simulink model "UAV_formacao"  (R2024b)
settings: Solver=VariableStepAuto  StartTime=0.0  StopTime=tsim  RelTol=1e-3
values from neighbouring files (symbols this model uses):
  A = [ybb, yp+(w0/u0), yr-(u0/u0), g*cos(tt0)/u0 ... (first row only)    [init.m]    (also in new_A_B_integrativos.m = [A, zeros, zeros]; new_A_B_lambda.m = [A, zeros])
  B = [Yda, Ydr ... (first row only)    [init.m]    (also in new_A_B_integrativos.m = [B; new_line_bb; new_line_lambda]; new_A_B_lambda.m = [B; new_line_B])
  C = [0,1,0,0,0;0,0,1,0,0;-1,0,0,0,1;]    [main.m]    (also in untitled2.m = diag([1,1,1,1]))
  E0_f = P_f(1)    [main.m]
  E0_l = P_l(1)    [main.m]
  freq_amost = 100    [main.m]
  gg0 = 0    [Grupo3RP1.m]    (also in all_values.m; init.m; main.m; new_A_B_lambda.m)
  H = 0.44    [main.m]
  K = lqr(A_temp,B_temp,Q,R)    [K_lqr.m]    (also in k_finder.m = [0,0,0,0; main.m = K_lqr(A,B); untitled2.m = [0,0,0.229,0])
  L = lqe(A,G,C,Qe,Re)    [L_estim.m]    (also in k_finder.m = linspace(0,100,9999); main.m = L_estim(A,C))
  N0_f = P_f(2)    [main.m]
  N0_l = P_l(2)    [main.m]
  ref = [deg2rad(0), deg2rad(90)]    [main.m]
  sample_time = 1/freq_amost    (= 0.01)    [main.m]
  sample_time_gps = 1/freq_amos_gps    (= 0.2)    [main.m]
  t_slope = 10    [main.m]
  t_start = 20    [main.m]
  t_still = 50    [main.m]
  tt0 = gg0 + aa0    (= -3.65)    [Grupo3RP1.m]    (also in all_values.m; init.m; main.m; new_A_B_lambda.m)
  u0 = u0*0.51444    (= 27.985536)    [Grupo3RP1.m]    (also in all_values.m; init.m = [da0, dr0]; main.m; untitled2.m)
  Vwind = 3    [main.m]
  x0 = min(y_diff.signals.values)    [graficos_formacao.m]    (also in init.m = [0,0,0,0]; new_A_B_lambda.m = [0,0,0,0,0]')
libraries: simulink x24
settings Model: Creator=ruben  LastModifiedBy=quico
settings DataIOCC: ReturnWorkspaceOutputs=off

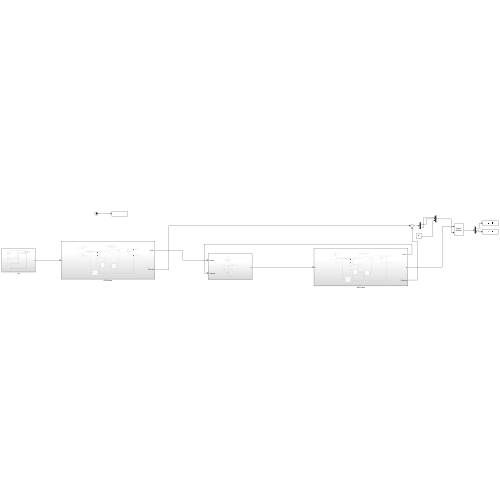
[thumbnail: Simulink's stored preview of the top-level diagram]
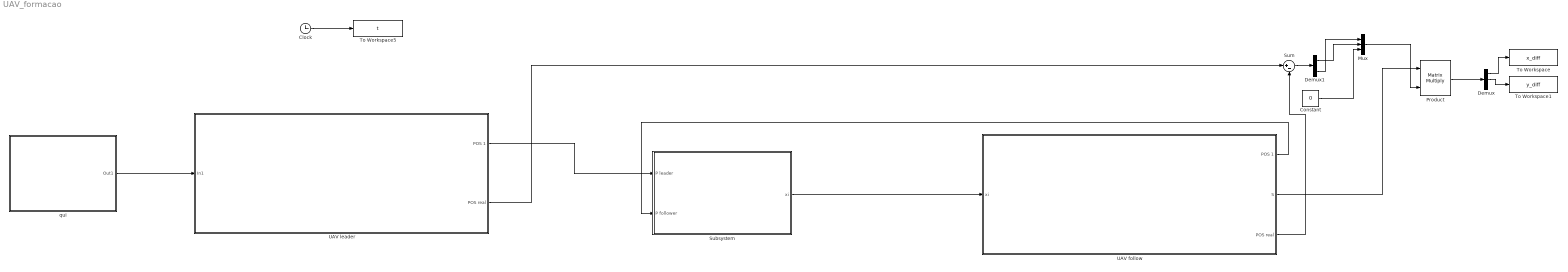
== system UAV_formacao ==
  " qui" : Subsystem
  Clock : Clock
  Constant : Constant  Value=0
  Demux : Demux  Outputs=3
  Demux1 : Demux  Outputs=2
  Mux : Mux  Inputs=3
  Product : Product  Multiplication=Matrix(*)
  Subsystem : Subsystem
  Sum : Sum  Inputs=|+-
  To Workspace : ToWorkspace  VariableName=x_diff  SaveFormat=Structure With Time  SampleTime=-1
  To Workspace1 : ToWorkspace  VariableName=y_diff  SaveFormat=Structure With Time  SampleTime=-1
  To Workspace5 : ToWorkspace  VariableName=t  SampleTime=-1
  UAV follow : Subsystem
  UAV leader : Subsystem
  wires:
  Clock/1 -> To Workspace5/1
  UAV leader/1(POS 1) -> Subsystem/1(P leader)
  UAV follow/1(POS 1) -> Subsystem/2(P follower)
  Subsystem/1(xi) -> UAV follow/1(xi)
  " qui"/1(Out1) -> UAV leader/1(In1)
  Product/1 -> Demux/1
  Demux/2 -> To Workspace1/1
  Demux/1 -> To Workspace/1
  Mux/1 -> Product/2
  UAV follow/2(S) -> Product/1
  Sum/1 -> Demux1/1
  Demux1/1 -> Mux/2
  Demux1/2 -> Mux/1
  Constant/1 -> Mux/3
  UAV leader/2(POS real) -> Sum/1
  UAV follow/3(POS real) -> Sum/2

== system UAV_formacao/ qui ==
  Ramp : simulink/Sources/Ramp  slope=ref(2)/t_slope  start=t_start  InitialOutput=0
  Ramp1 : simulink/Sources/Ramp  slope=-ref(2)/t_slope  start=t_start+t_slope  InitialOutput=0
  Ramp2 : simulink/Sources/Ramp  slope=-ref(2)/t_slope  start=t_start+t_slope+t_still  InitialOutput=0
  Ramp3 : simulink/Sources/Ramp  slope=ref(2)/t_slope  start=t_start+t_slope+t_still+t_slope  InitialOutput=0
  Sum1 : Sum  Inputs=|++++
  Out1 : Outport
  wires:
  Sum1/1 -> Out1/1
  Ramp/1 -> Sum1/1
  Ramp1/1 -> Sum1/2
  Ramp2/1 -> Sum1/3
  Ramp3/1 -> Sum1/4

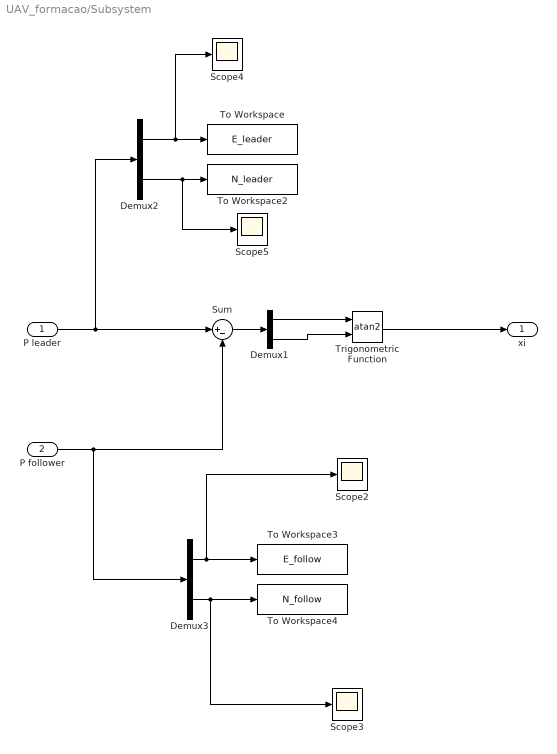
== system UAV_formacao/Subsystem ==
  P leader : Inport
  P follower : Inport  Port=2
  Demux1 : Demux  Outputs=2
  Demux2 : Demux  Outputs=2
  Demux3 : Demux  Outputs=2
  Scope{2..5} (4 alike) : Scope
  Sum : Sum  Inputs=|+-
  To Workspace : ToWorkspace  VariableName=E_leader  SaveFormat=Structure With Time  SampleTime=-1
  To Workspace2 : ToWorkspace  VariableName=N_leader  SaveFormat=Structure With Time  SampleTime=-1
  To Workspace3 : ToWorkspace  VariableName=E_follow  SaveFormat=Structure With Time  SampleTime=-1
  To Workspace4 : ToWorkspace  VariableName=N_follow  SaveFormat=Structure With Time  SampleTime=-1
  Trigonometric Function : Trigonometry  Operator=atan2
  xi : Outport
  wires:
  P leader/1 -> Demux2/1, Sum/1
  P follower/1 -> Demux3/1, Sum/2
  Demux2/1 -> Scope4/1, To Workspace/1
  Demux2/2 -> Scope5/1, To Workspace2/1
  Demux3/2 -> Scope3/1, To Workspace4/1
  Demux3/1 -> Scope2/1, To Workspace3/1
  Sum/1 -> Demux1/1
  Demux1/1 -> Trigonometric Function/1
  Demux1/2 -> Trigonometric Function/2
  Trigonometric Function/1 -> xi/1

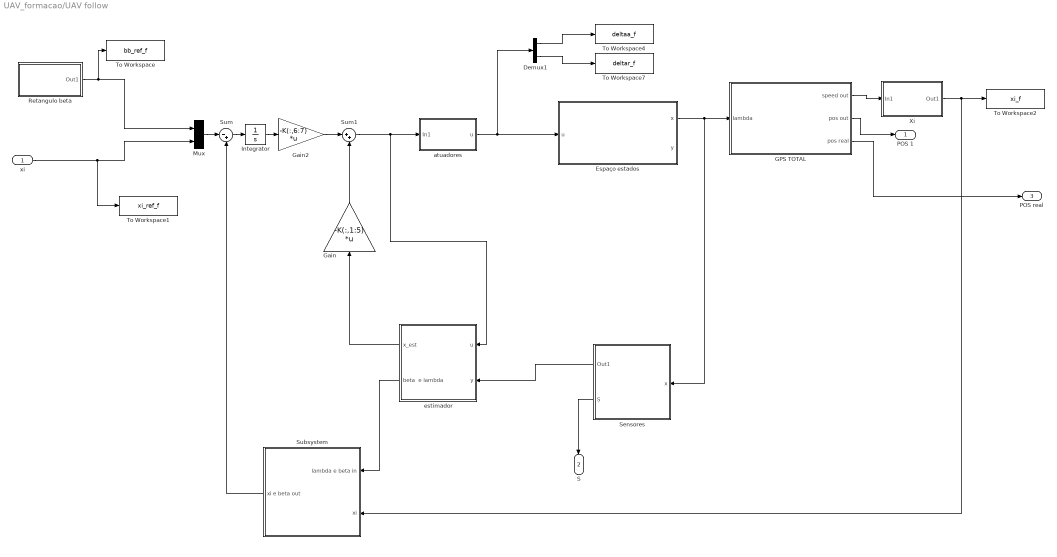
== system UAV_formacao/UAV follow ==
  xi : Inport
  Demux1 : Demux  Outputs=2
  Espaço estados : Subsystem
  GPS TOTAL : Subsystem
  Gain : Gain  Gain=-K(:,1:5)  Multiplication=Matrix(K*u)
  Gain2 : Gain  Gain=-K(:,6:7)  Multiplication=Matrix(K*u)
  Integrator : Integrator  InitialCondition=[0,0]
  Mux : Mux  Inputs=2
  Retangulo beta : Subsystem
  Sensores : Subsystem
  Subsystem : Subsystem
  Sum : Sum  Inputs=|-+
  Sum1 : Sum  Inputs=|++
  To Workspace : ToWorkspace  VariableName=bb_ref_f  SampleTime=-1
  To Workspace1 : ToWorkspace  VariableName=xi_ref_f  SampleTime=-1
  To Workspace2 : ToWorkspace  VariableName=xi_f  SaveFormat=Structure With Time  SampleTime=-1
  To Workspace4 : ToWorkspace  VariableName=deltaa_f  SampleTime=-1
  To Workspace7 : ToWorkspace  VariableName=deltar_f  SampleTime=-1
  Xi : Subsystem
  atuadores : Subsystem
  estimador : Subsystem
  POS 1 : Outport
  S : Outport  Port=2
  POS real : Outport  Port=3
  wires:
  Retangulo beta/1(Out1) -> To Workspace/1, Mux/1
  estimador/2(beta  e lambda) -> Subsystem/1(lambda e beta in)
  Gain/1 -> Sum1/2
  Sensores/1(Out1) -> estimador/2(y)
  estimador/1(x_est) -> Gain/1
  xi/1 -> To Workspace1/1, Mux/2
  Mux/1 -> Sum/1
  Sum/1 -> Integrator/1
  Integrator/1 -> Gain2/1
  Sum1/1 -> estimador/1(u), atuadores/1(In1)
  atuadores/1(u) -> Espaço estados/1(u), Demux1/1
  Subsystem/1(xi e beta out) -> Sum/2
  Gain2/1 -> Sum1/1
  Demux1/1 -> To Workspace4/1
  Demux1/2 -> To Workspace7/1
  GPS TOTAL/2(pos out) -> POS 1/1
  GPS TOTAL/1(speed out) -> Xi/1(In1)
  Xi/1(Out1) -> Subsystem/2(xi), To Workspace2/1
  Espaço estados/1(x) -> Sensores/1(x), GPS TOTAL/1(lambda)
  Sensores/2(S) -> S/1
  GPS TOTAL/3(pos real) -> POS real/1

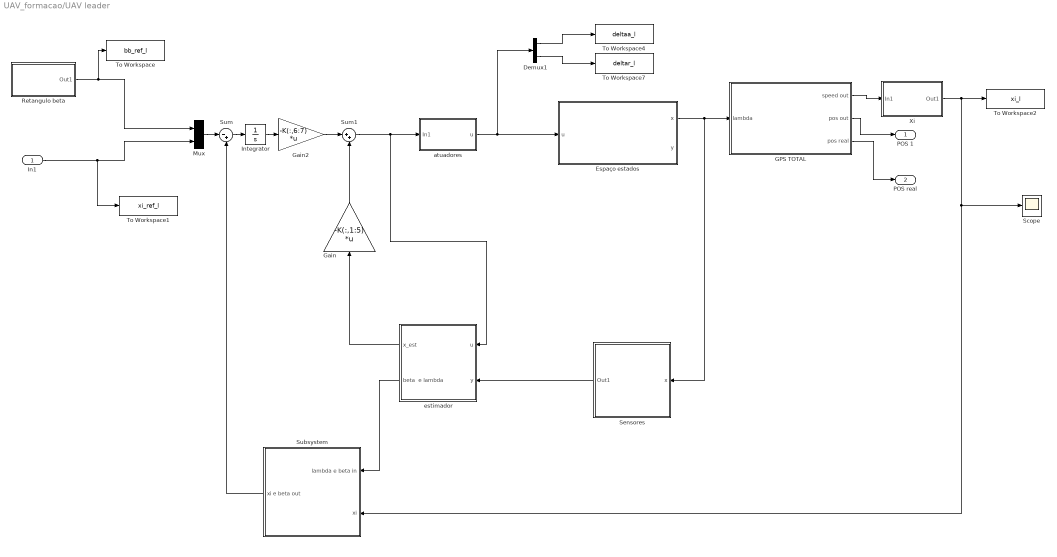
== system UAV_formacao/UAV leader ==
  In1 : Inport
  Demux1 : Demux  Outputs=2
  Espaço estados : Subsystem
  GPS TOTAL : Subsystem
  Gain : Gain  Gain=-K(:,1:5)  Multiplication=Matrix(K*u)
  Gain2 : Gain  Gain=-K(:,6:7)  Multiplication=Matrix(K*u)
  Integrator : Integrator  InitialCondition=[0,0]
  Mux : Mux  Inputs=2
  Retangulo beta : Subsystem
  Scope : Scope
  Sensores : Subsystem
  Subsystem : Subsystem
  Sum : Sum  Inputs=|-+
  Sum1 : Sum  Inputs=|++
  To Workspace : ToWorkspace  VariableName=bb_ref_l  SampleTime=-1
  To Workspace1 : ToWorkspace  VariableName=xi_ref_l  SampleTime=-1
  To Workspace2 : ToWorkspace  VariableName=xi_l  SaveFormat=Structure With Time  SampleTime=-1
  To Workspace4 : ToWorkspace  VariableName=deltaa_l  SampleTime=-1
  To Workspace7 : ToWorkspace  VariableName=deltar_l  SampleTime=-1
  Xi : Subsystem
  atuadores : Subsystem
  estimador : Subsystem
  POS 1 : Outport
  POS real : Outport  Port=2
  wires:
  Retangulo beta/1(Out1) -> To Workspace/1, Mux/1
  estimador/2(beta  e lambda) -> Subsystem/1(lambda e beta in)
  Gain/1 -> Sum1/2
  Sensores/1(Out1) -> estimador/2(y)
  estimador/1(x_est) -> Gain/1
  In1/1 -> To Workspace1/1, Mux/2
  Mux/1 -> Sum/1
  Sum/1 -> Integrator/1
  Integrator/1 -> Gain2/1
  Sum1/1 -> estimador/1(u), atuadores/1(In1)
  atuadores/1(u) -> Espaço estados/1(u), Demux1/1
  Subsystem/1(xi e beta out) -> Sum/2
  Gain2/1 -> Sum1/1
  Demux1/1 -> To Workspace4/1
  Demux1/2 -> To Workspace7/1
  GPS TOTAL/2(pos out) -> POS 1/1
  GPS TOTAL/1(speed out) -> Xi/1(In1)
  Xi/1(Out1) -> Scope/1, Subsystem/2(xi), To Workspace2/1
  Espaço estados/1(x) -> Sensores/1(x), GPS TOTAL/1(lambda)
  GPS TOTAL/3(pos real) -> POS real/1

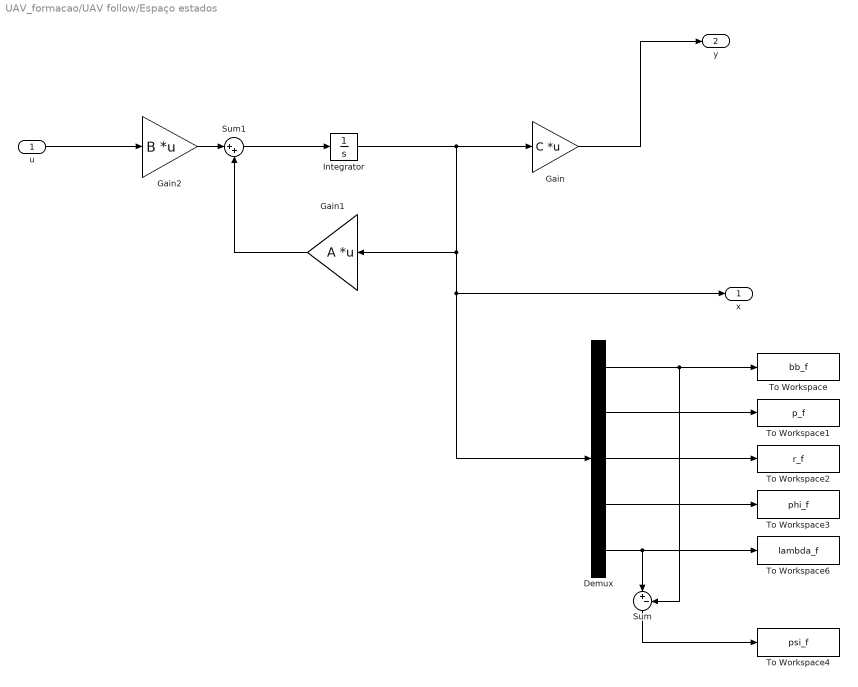
== system UAV_formacao/UAV follow/Espaço estados ==
  u : Inport
  Demux : Demux  Outputs=5
  Gain : Gain  Gain=C  Multiplication=Matrix(K*u)
  Gain1 : Gain  Gain=A  Multiplication=Matrix(K*u)
  Gain2 : Gain  Gain=B  Multiplication=Matrix(K*u)
  Integrator : Integrator  InitialCondition=x0
  Sum : Sum  Inputs=|+-
  Sum1 : Sum  Inputs=|++
  To Workspace : ToWorkspace  VariableName=bb_f  SampleTime=-1
  To Workspace1 : ToWorkspace  VariableName=p_f  SampleTime=-1
  To Workspace2 : ToWorkspace  VariableName=r_f  SampleTime=-1
  To Workspace3 : ToWorkspace  VariableName=phi_f  SampleTime=-1
  To Workspace4 : ToWorkspace  VariableName=psi_f  SampleTime=-1
  To Workspace6 : ToWorkspace  VariableName=lambda_f  SampleTime=-1
  x : Outport
  y : Outport  Port=2
  wires:
  u/1 -> Gain2/1
  Sum1/1 -> Integrator/1
  Demux/4 -> To Workspace3/1
  Demux/3 -> To Workspace2/1
  Demux/1 -> Sum/2, To Workspace/1
  Demux/2 -> To Workspace1/1
  Demux/5 -> Sum/1, To Workspace6/1
  Gain2/1 -> Sum1/1
  Integrator/1 -> Gain1/1, x/1, Demux/1, Gain/1
  Gain1/1 -> Sum1/2
  Gain/1 -> y/1
  Sum/1 -> To Workspace4/1

== system UAV_formacao/UAV follow/GPS TOTAL ==
  lambda : Inport
  Cinematica : Subsystem
  GPS : Subsystem
  speed out : Outport
  pos out : Outport  Port=2
  pos real : Outport  Port=3
  wires:
  Cinematica/2(pos) -> pos real/1, GPS/2(pos)
  GPS/2(pos out) -> pos out/1
  Cinematica/1(speed) -> GPS/1(speed)
  lambda/1 -> Cinematica/1(lambda)
  GPS/1(speed out) -> speed out/1

== system UAV_formacao/UAV follow/Retangulo beta ==
  Sum1 : Sum  Inputs=|++
  beta : Step  Time=25  After=-ref(1)  SampleTime=0
  beta_1 : Step  Time=10  After=ref(1)  SampleTime=0
  Out1 : Outport
  wires:
  beta/1 -> Sum1/1
  beta_1/1 -> Sum1/2
  Sum1/1 -> Out1/1

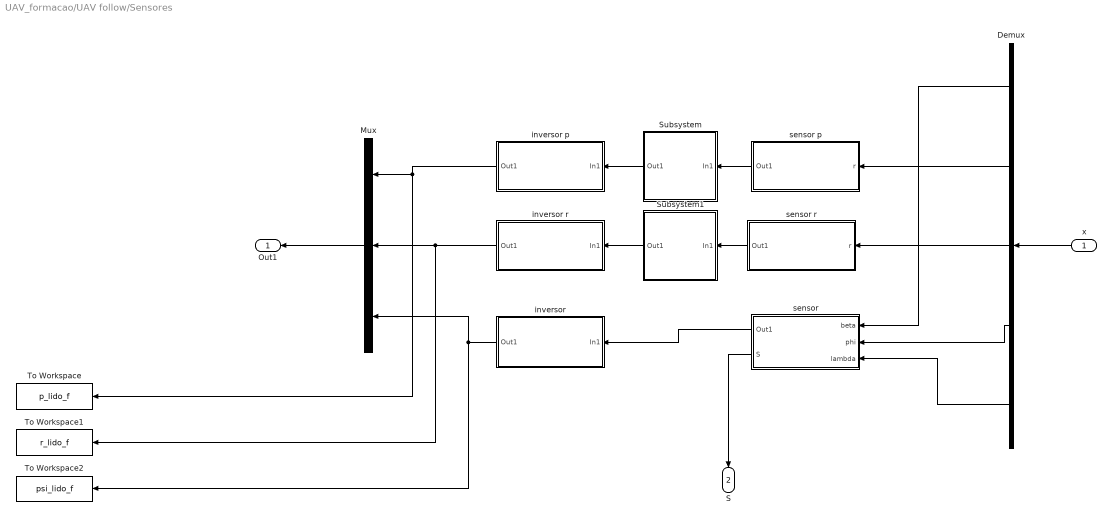
== system UAV_formacao/UAV follow/Sensores ==
  x : Inport
  Demux : Demux  Outputs=5
  Mux : Mux  Inputs=3
  Subsystem : Subsystem
  Subsystem1 : Subsystem
  To Workspace : ToWorkspace  VariableName=p_lido_f  SampleTime=-1
  To Workspace1 : ToWorkspace  VariableName=r_lido_f  SampleTime=-1
  To Workspace2 : ToWorkspace  VariableName=psi_lido_f  SampleTime=-1
  inversor : Subsystem
  inversor p : Subsystem
  inversor r : Subsystem
  sensor : Subsystem
  sensor p : Subsystem
  sensor r : Subsystem
  Out1 : Outport
  S : Outport  Port=2
  wires:
  inversor p/1(Out1) -> To Workspace/1, Mux/1
  Mux/1 -> Out1/1
  inversor r/1(Out1) -> To Workspace1/1, Mux/2
  x/1 -> Demux/1
  sensor/1(Out1) -> inversor/1(In1)
  inversor/1(Out1) -> To Workspace2/1, Mux/3
  Demux/2 -> sensor p/1(r)
  Demux/3 -> sensor r/1(r)
  Demux/1 -> sensor/1(beta)
  Demux/4 -> sensor/2(phi)
  Demux/5 -> sensor/3(lambda)
  Subsystem1/1(Out1) -> inversor r/1(In1)
  sensor r/1(Out1) -> Subsystem1/1(In1)
  sensor p/1(Out1) -> Subsystem/1(In1)
  Subsystem/1(Out1) -> inversor p/1(In1)
  sensor/2(S) -> S/1

== system UAV_formacao/UAV follow/Subsystem ==
  lambda e beta in : Inport
  xi : Inport  Port=2
  Demux : Demux  Outputs=2
  Mux1 : Mux  Inputs=2
  Sum2 : Sum  Inputs=|-+
  Sum3 : Sum  Inputs=|++
  xi e beta out : Outport
  wires:
  xi/1 -> Sum2/2
  Sum3/1 -> Mux1/2
  Demux/1 -> Mux1/1
  Mux1/1 -> xi e beta out/1
  lambda e beta in/1 -> Demux/1
  Demux/2 -> Sum2/1, Sum3/1
  Sum2/1 -> Sum3/2

== system UAV_formacao/UAV follow/Xi ==
  In1 : Inport
  Demux : Demux  Outputs=2
  Trigonometric Function : Trigonometry  Operator=atan2
  Out1 : Outport
  wires:
  Demux/1 -> Trigonometric Function/2
  Demux/2 -> Trigonometric Function/1
  Trigonometric Function/1 -> Out1/1
  In1/1 -> Demux/1

== system UAV_formacao/UAV follow/atuadores ==
  In1 : Inport
  Demux : Demux  Outputs=2
  Mux : Mux  Inputs=2
  Rate Limiter : RateLimiter  SampleTimeMode=inherited
  Rate Limiter1 : RateLimiter  SampleTimeMode=inherited
  Saturation : Saturate  UpperLimit=30*pi/180  LowerLimit=-30*pi/180
  Saturation1 : Saturate  UpperLimit=30*pi/180  LowerLimit=-30*pi/180
  Transfer Fcn : TransferFcn  Denominator=[0.04 1]
  Transfer Fcn1 : TransferFcn  Denominator=[0.04 1]
  Zero-Order Hold : ZeroOrderHold  SampleTime=1/100
  Zero-Order Hold1 : ZeroOrderHold  SampleTime=1/100
  u : Outport
  wires:
  In1/1 -> Demux/1
  Mux/1 -> u/1
  Demux/1 -> Zero-Order Hold/1  "deltaa"
  Demux/2 -> Zero-Order Hold1/1  "deltar"
  Transfer Fcn1/1 -> Mux/2
  Transfer Fcn/1 -> Mux/1
  Rate Limiter/1 -> Transfer Fcn/1
  Rate Limiter1/1 -> Transfer Fcn1/1
  Saturation1/1 -> Rate Limiter1/1
  Saturation/1 -> Rate Limiter/1
  Zero-Order Hold/1 -> Saturation/1
  Zero-Order Hold1/1 -> Saturation1/1

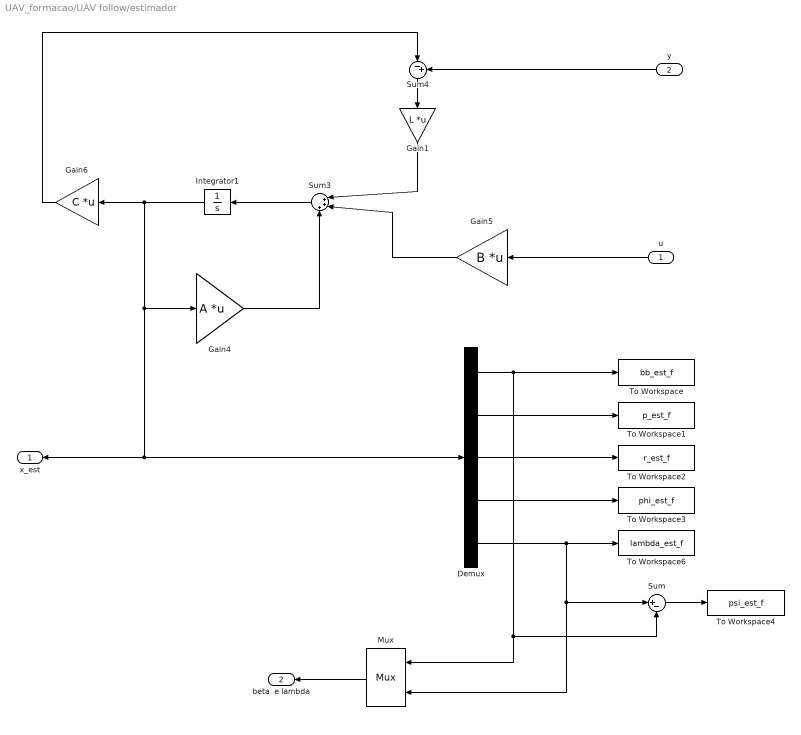
== system UAV_formacao/UAV follow/estimador ==
  u : Inport
  y : Inport  Port=2
  Demux : Demux  Outputs=5
  Gain1 : Gain  Gain=L  Multiplication=Matrix(K*u)
  Gain4 : Gain  Gain=A  Multiplication=Matrix(K*u)
  Gain5 : Gain  Gain=B  Multiplication=Matrix(K*u)
  Gain6 : Gain  Gain=C  Multiplication=Matrix(K*u)
  Integrator1 : Integrator  InitialCondition=x0
  Mux : Mux  Inputs=2
      settings: DisplayOption=signals
  Sum : Sum  Inputs=|+-
  Sum3 : Sum  Inputs=|+++
  Sum4 : Sum  Inputs=|-+
  To Workspace : ToWorkspace  VariableName=bb_est_f  SampleTime=-1
  To Workspace1 : ToWorkspace  VariableName=p_est_f  SampleTime=-1
  To Workspace2 : ToWorkspace  VariableName=r_est_f  SampleTime=-1
  To Workspace3 : ToWorkspace  VariableName=phi_est_f  SampleTime=-1
  To Workspace4 : ToWorkspace  VariableName=psi_est_f  SampleTime=-1
  To Workspace6 : ToWorkspace  VariableName=lambda_est_f  SampleTime=-1
  x_est : Outport
  beta  e lambda : Outport  Port=2
  wires:
  Demux/5 -> Sum/1, Mux/2, To Workspace6/1
  Demux/2 -> To Workspace1/1
  Demux/3 -> To Workspace2/1
  Demux/4 -> To Workspace3/1
  Demux/1 -> Sum/2, Mux/1, To Workspace/1
  Integrator1/1 -> Demux/1, x_est/1, Gain4/1, Gain6/1
  Sum3/1 -> Integrator1/1
  u/1 -> Gain5/1
  Gain4/1 -> Sum3/3
  y/1 -> Sum4/2
  Gain6/1 -> Sum4/1
  Gain5/1 -> Sum3/2
  Mux/1 -> beta  e lambda/1
  Sum4/1 -> Gain1/1
  Gain1/1 -> Sum3/1
  Sum/1 -> To Workspace4/1

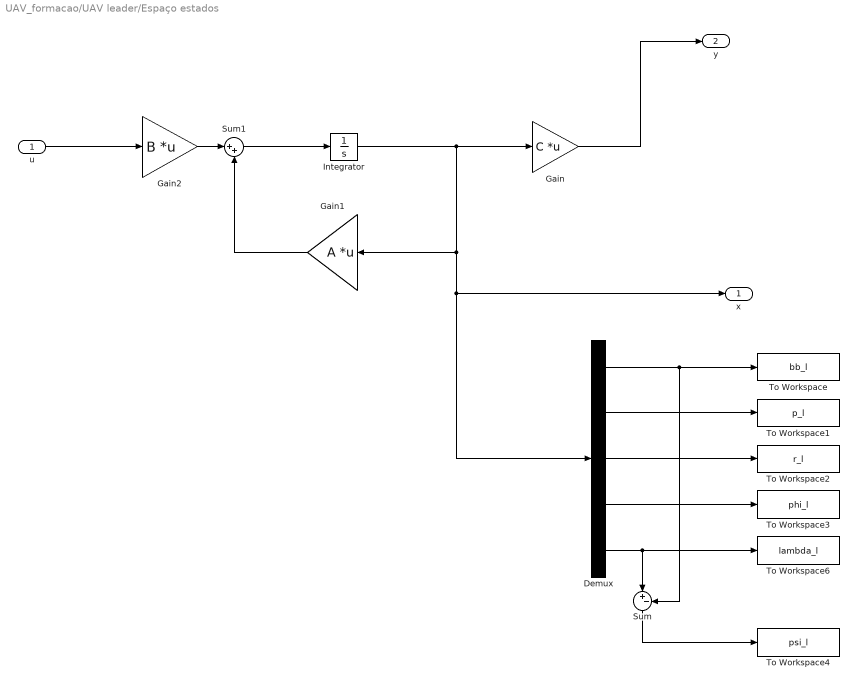
== system UAV_formacao/UAV leader/Espaço estados ==
  u : Inport
  Demux : Demux  Outputs=5
  Gain : Gain  Gain=C  Multiplication=Matrix(K*u)
  Gain1 : Gain  Gain=A  Multiplication=Matrix(K*u)
  Gain2 : Gain  Gain=B  Multiplication=Matrix(K*u)
  Integrator : Integrator  InitialCondition=x0
  Sum : Sum  Inputs=|+-
  Sum1 : Sum  Inputs=|++
  To Workspace : ToWorkspace  VariableName=bb_l  SampleTime=-1
  To Workspace1 : ToWorkspace  VariableName=p_l  SampleTime=-1
  To Workspace2 : ToWorkspace  VariableName=r_l  SampleTime=-1
  To Workspace3 : ToWorkspace  VariableName=phi_l  SampleTime=-1
  To Workspace4 : ToWorkspace  VariableName=psi_l  SampleTime=-1
  To Workspace6 : ToWorkspace  VariableName=lambda_l  SampleTime=-1
  x : Outport
  y : Outport  Port=2
  wires:
  u/1 -> Gain2/1
  Sum1/1 -> Integrator/1
  Demux/4 -> To Workspace3/1
  Demux/3 -> To Workspace2/1
  Demux/1 -> Sum/2, To Workspace/1
  Demux/2 -> To Workspace1/1
  Demux/5 -> Sum/1, To Workspace6/1
  Gain2/1 -> Sum1/1
  Integrator/1 -> Gain1/1, x/1, Demux/1, Gain/1
  Gain1/1 -> Sum1/2
  Gain/1 -> y/1
  Sum/1 -> To Workspace4/1

== system UAV_formacao/UAV leader/GPS TOTAL ==
  lambda : Inport
  Cinematica : Subsystem
  GPS : Subsystem
  speed out : Outport
  pos out : Outport  Port=2
  pos real : Outport  Port=3
  wires:
  Cinematica/2(pos) -> pos real/1, GPS/2(pos)
  GPS/2(pos out) -> pos out/1
  Cinematica/1(speed) -> GPS/1(speed)
  lambda/1 -> Cinematica/1(lambda)
  GPS/1(speed out) -> speed out/1

== system UAV_formacao/UAV leader/Retangulo beta ==
  Sum1 : Sum  Inputs=|++
  beta : Step  Time=25  After=-ref(1)  SampleTime=0
  beta_1 : Step  Time=10  After=ref(1)  SampleTime=0
  Out1 : Outport
  wires:
  beta/1 -> Sum1/1
  beta_1/1 -> Sum1/2
  Sum1/1 -> Out1/1

== system UAV_formacao/UAV leader/Sensores ==
  x : Inport
  Demux : Demux  Outputs=5
  Mux : Mux  Inputs=3
  Subsystem : Subsystem
  Subsystem1 : Subsystem
  To Workspace : ToWorkspace  VariableName=p_lido_l  SampleTime=-1
  To Workspace1 : ToWorkspace  VariableName=r_lido_l  SampleTime=-1
  To Workspace2 : ToWorkspace  VariableName=psi_lido_l  SampleTime=-1
  inversor : Subsystem
  inversor p : Subsystem
  inversor r : Subsystem
  sensor : Subsystem
  sensor p : Subsystem
  sensor r : Subsystem
  Out1 : Outport
  wires:
  inversor p/1(Out1) -> To Workspace/1, Mux/1
  Mux/1 -> Out1/1
  inversor r/1(Out1) -> To Workspace1/1, Mux/2
  x/1 -> Demux/1
  sensor/1(Out1) -> inversor/1(In1)
  inversor/1(Out1) -> To Workspace2/1, Mux/3
  Demux/2 -> sensor p/1(r)
  Demux/3 -> sensor r/1(r)
  Demux/1 -> sensor/1(beta)
  Demux/4 -> sensor/2(phi)
  Demux/5 -> sensor/3(lambda)
  Subsystem1/1(Out1) -> inversor r/1(In1)
  sensor r/1(Out1) -> Subsystem1/1(In1)
  sensor p/1(Out1) -> Subsystem/1(In1)
  Subsystem/1(Out1) -> inversor p/1(In1)

== system UAV_formacao/UAV leader/Subsystem ==
  lambda e beta in : Inport
  xi : Inport  Port=2
  Demux : Demux  Outputs=2
  Mux1 : Mux  Inputs=2
  Sum2 : Sum  Inputs=|-+
  Sum3 : Sum  Inputs=|++
  xi e beta out : Outport
  wires:
  xi/1 -> Sum2/2
  Sum3/1 -> Mux1/2
  Demux/1 -> Mux1/1
  Mux1/1 -> xi e beta out/1
  lambda e beta in/1 -> Demux/1
  Demux/2 -> Sum2/1, Sum3/1
  Sum2/1 -> Sum3/2

== system UAV_formacao/UAV leader/Xi ==
  In1 : Inport
  Demux : Demux  Outputs=2
  Trigonometric Function : Trigonometry  Operator=atan2
  Out1 : Outport
  wires:
  Demux/1 -> Trigonometric Function/2
  Demux/2 -> Trigonometric Function/1
  Trigonometric Function/1 -> Out1/1
  In1/1 -> Demux/1

== system UAV_formacao/UAV leader/atuadores ==
  In1 : Inport
  Demux : Demux  Outputs=2
  Mux : Mux  Inputs=2
  Rate Limiter : RateLimiter  SampleTimeMode=inherited
  Rate Limiter1 : RateLimiter  SampleTimeMode=inherited
  Saturation : Saturate  UpperLimit=30*pi/180  LowerLimit=-30*pi/180
  Saturation1 : Saturate  UpperLimit=30*pi/180  LowerLimit=-30*pi/180
  Transfer Fcn : TransferFcn  Denominator=[0.04 1]
  Transfer Fcn1 : TransferFcn  Denominator=[0.04 1]
  Zero-Order Hold : ZeroOrderHold  SampleTime=1/100
  Zero-Order Hold1 : ZeroOrderHold  SampleTime=1/100
  u : Outport
  wires:
  In1/1 -> Demux/1
  Mux/1 -> u/1
  Demux/1 -> Zero-Order Hold/1  "deltaa"
  Demux/2 -> Zero-Order Hold1/1  "deltar"
  Transfer Fcn1/1 -> Mux/2
  Transfer Fcn/1 -> Mux/1
  Rate Limiter/1 -> Transfer Fcn/1
  Rate Limiter1/1 -> Transfer Fcn1/1
  Saturation1/1 -> Rate Limiter1/1
  Saturation/1 -> Rate Limiter/1
  Zero-Order Hold/1 -> Saturation/1
  Zero-Order Hold1/1 -> Saturation1/1

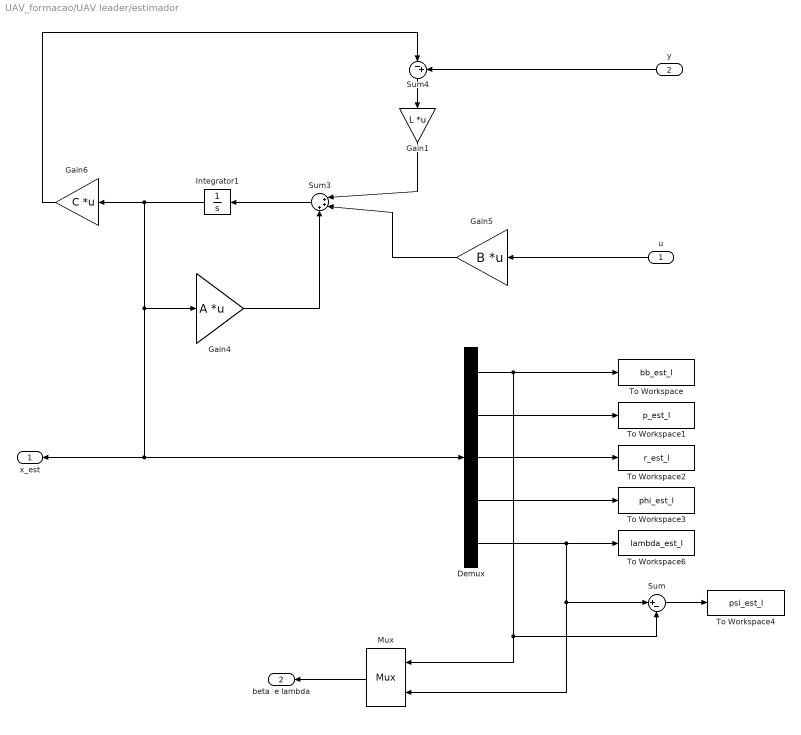
== system UAV_formacao/UAV leader/estimador ==
  u : Inport
  y : Inport  Port=2
  Demux : Demux  Outputs=5
  Gain1 : Gain  Gain=L  Multiplication=Matrix(K*u)
  Gain4 : Gain  Gain=A  Multiplication=Matrix(K*u)
  Gain5 : Gain  Gain=B  Multiplication=Matrix(K*u)
  Gain6 : Gain  Gain=C  Multiplication=Matrix(K*u)
  Integrator1 : Integrator  InitialCondition=x0
  Mux : Mux  Inputs=2
      settings: DisplayOption=signals
  Sum : Sum  Inputs=|+-
  Sum3 : Sum  Inputs=|+++
  Sum4 : Sum  Inputs=|-+
  To Workspace : ToWorkspace  VariableName=bb_est_l  SampleTime=-1
  To Workspace1 : ToWorkspace  VariableName=p_est_l  SampleTime=-1
  To Workspace2 : ToWorkspace  VariableName=r_est_l  SampleTime=-1
  To Workspace3 : ToWorkspace  VariableName=phi_est_l  SampleTime=-1
  To Workspace4 : ToWorkspace  VariableName=psi_est_l  SampleTime=-1
  To Workspace6 : ToWorkspace  VariableName=lambda_est_l  SampleTime=-1
  x_est : Outport
  beta  e lambda : Outport  Port=2
  wires:
  Demux/5 -> Sum/1, Mux/2, To Workspace6/1
  Demux/2 -> To Workspace1/1
  Demux/3 -> To Workspace2/1
  Demux/4 -> To Workspace3/1
  Demux/1 -> Sum/2, Mux/1, To Workspace/1
  Integrator1/1 -> Demux/1, x_est/1, Gain4/1, Gain6/1
  Sum3/1 -> Integrator1/1
  u/1 -> Gain5/1
  Gain4/1 -> Sum3/3
  y/1 -> Sum4/2
  Gain6/1 -> Sum4/1
  Gain5/1 -> Sum3/2
  Mux/1 -> beta  e lambda/1
  Sum4/1 -> Gain1/1
  Gain1/1 -> Sum3/1
  Sum/1 -> To Workspace4/1

== system UAV_formacao/UAV follow/GPS TOTAL/Cinematica ==
  lambda : Inport
  Constant1 : Constant  Value=gg0
  Constant2 : Constant  Value=u0
  Constant3 : Constant  Value=Vwind
  Demux : Demux  Outputs=5
  Integrator : Integrator  InitialCondition=E0_f
  Integrator1 : Integrator  InitialCondition=N0_f
  Mux1 : Mux  Inputs=2
  Mux2 : Mux  Inputs=2
  Product2 : Product
  Product3 : Product
  Subsystem : Subsystem
  Subsystem1 : Subsystem
  Sum : Sum  Inputs=|+-
  speed : Outport
  pos : Outport  Port=2
  wires:
  Constant2/1 -> Product3/2, Product2/1
  Product3/1 -> Mux2/2, Integrator/1
  Product2/1 -> Sum/1
  Constant3/1 -> Sum/2
  Sum/1 -> Mux2/1, Integrator1/1
  Integrator/1 -> Mux1/1
  Integrator1/1 -> Mux1/2
  Mux2/1 -> speed/1
  Mux1/1 -> pos/1
  Subsystem/1(Out1) -> Product3/1
  Constant1/1 -> Subsystem/2(In2), Subsystem1/1(In2)
  Subsystem1/1(Out1) -> Product2/2
  lambda/1 -> Demux/1
  Demux/5 -> Subsystem/1(In1), Subsystem1/2(In1)

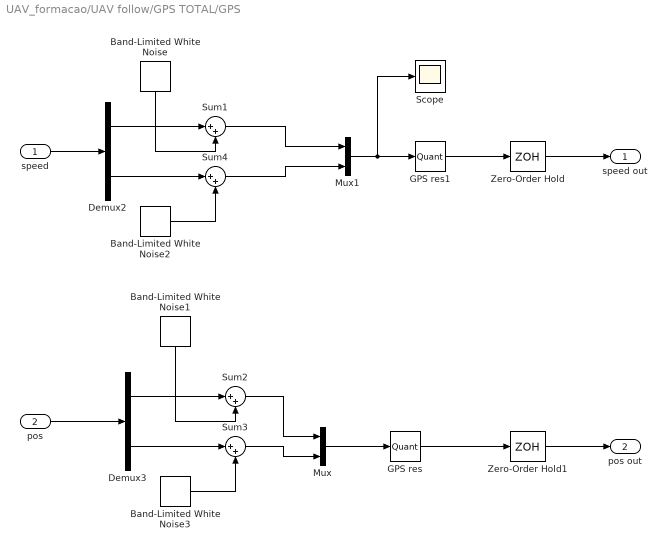
== system UAV_formacao/UAV follow/GPS TOTAL/GPS ==
  speed : Inport
  pos : Inport  Port=2
  Band-Limited White Noise : simulink/Sources/Band-Limited White Noise  Cov=sample_time_gps*0.1*0.1  Ts=sample_time_gps  seed=[13]
  Band-Limited White Noise1 : simulink/Sources/Band-Limited White Noise  Cov=sample_time_gps*2.5*2.5  Ts=sample_time_gps  seed=[15]
  Band-Limited White Noise2 : simulink/Sources/Band-Limited White Noise  Cov=sample_time_gps*0.1*0.1  Ts=sample_time_gps  seed=[14]
  Band-Limited White Noise3 : simulink/Sources/Band-Limited White Noise  Cov=sample_time_gps*2.5*2.5  Ts=sample_time_gps  seed=[16]
  Demux2 : Demux  Outputs=2
  Demux3 : Demux  Outputs=2
  GPS res : Quantizer
  GPS res1 : Quantizer  QuantizationInterval=0.01
  Mux : Mux  Inputs=2
  Mux1 : Mux  Inputs=2
  Scope : Scope
  Sum{1..4} (4 alike) : Sum  Inputs=|++
  Zero-Order Hold : ZeroOrderHold  SampleTime=sample_time_gps
  Zero-Order Hold1 : ZeroOrderHold  SampleTime=sample_time_gps
  speed out : Outport
  pos out : Outport  Port=2
  wires:
  Mux/1 -> GPS res/1
  GPS res/1 -> Zero-Order Hold1/1
  GPS res1/1 -> Zero-Order Hold/1
  Mux1/1 -> Scope/1, GPS res1/1
  speed/1 -> Demux2/1
  Demux2/1 -> Sum1/1
  Demux2/2 -> Sum4/1
  Band-Limited White Noise/1 -> Sum1/2
  Band-Limited White Noise2/1 -> Sum4/2
  Demux3/2 -> Sum3/1
  pos/1 -> Demux3/1
  Band-Limited White Noise3/1 -> Sum3/2
  Demux3/1 -> Sum2/1
  Band-Limited White Noise1/1 -> Sum2/2
  Sum2/1 -> Mux/1
  Sum3/1 -> Mux/2
  Sum4/1 -> Mux1/2
  Sum1/1 -> Mux1/1
  Zero-Order Hold/1 -> speed out/1
  Zero-Order Hold1/1 -> pos out/1

== system UAV_formacao/UAV follow/Sensores/Subsystem ==
  In1 : Inport
  Band-Limited White Noise : simulink/Sources/Band-Limited White Noise  Cov=[sample_time*(2*(5/(2^12)))^2]  Ts=sample_time  seed=[1]
  Quantizer : Quantizer  QuantizationInterval=5/(2^12)
  Saturation : Saturate  UpperLimit=5  LowerLimit=0
  Sum : Sum  Inputs=|++
  Out1 : Outport
  wires:
  In1/1 -> Sum/1
  Saturation/1 -> Out1/1
  Band-Limited White Noise/1 -> Sum/2
  Quantizer/1 -> Saturation/1
  Sum/1 -> Quantizer/1

== system UAV_formacao/UAV follow/Sensores/Subsystem1 ==
  In1 : Inport
  Band-Limited White Noise : simulink/Sources/Band-Limited White Noise  Cov=[sample_time*(2*(5/(2^12)))^2]  Ts=sample_time  seed=[2]
  Quantizer : Quantizer  QuantizationInterval=5/(2^12)
  Saturation : Saturate  UpperLimit=5  LowerLimit=0
  Sum : Sum  Inputs=|++
  Out1 : Outport
  wires:
  In1/1 -> Sum/1
  Saturation/1 -> Out1/1
  Band-Limited White Noise/1 -> Sum/2
  Quantizer/1 -> Saturation/1
  Sum/1 -> Quantizer/1

== system UAV_formacao/UAV follow/Sensores/inversor ==
  In1 : Inport
  Band-Limited White Noise1 : simulink/Sources/Band-Limited White Noise  Cov=[0.005*0.005*freq_amost]  Ts=freq_amost  seed=[11]
  Band-Limited White Noise2 : simulink/Sources/Band-Limited White Noise  Cov=[0.005*0.005*sample_time]  Ts=sample_time  seed=[12]
  Demux : Demux  Outputs=3
  Gain : Gain  Gain=-1
  Quantizer : Quantizer  QuantizationInterval=0.005
  Quantizer1 : Quantizer  QuantizationInterval=0.005
  Saturation : Saturate  UpperLimit=8  LowerLimit=-8
  Saturation1 : Saturate  UpperLimit=8  LowerLimit=-8
  Sum : Sum  Inputs=|++
  Sum1 : Sum  Inputs=|++
  Trigonometric Function : Trigonometry  Operator=atan2
  Out1 : Outport
  wires:
  Band-Limited White Noise1/1 -> Sum/2
  Band-Limited White Noise2/1 -> Sum1/2
  Sum/1 -> Quantizer/1
  Sum1/1 -> Quantizer1/1
  Demux/1 -> Sum/1
  Trigonometric Function/1 -> Out1/1
  In1/1 -> Demux/1
  Demux/2 -> Sum1/1
  Gain/1 -> Trigonometric Function/1
  Saturation1/1 -> Gain/1
  Quantizer1/1 -> Saturation1/1
  Quantizer/1 -> Saturation/1
  Saturation/1 -> Trigonometric Function/2

== system UAV_formacao/UAV follow/Sensores/inversor p ==
  In1 : Inport
  Constant : Constant  Value=-1250/3
  Gain3 : Gain  Gain=(300-(-300))/(4.3-0.7)
  Gain5 : Gain  Gain=pi/180
  Sum : Sum  Inputs=|++
  Out1 : Outport
  wires:
  In1/1 -> Gain3/1
  Gain5/1 -> Out1/1
  Gain3/1 -> Sum/1
  Sum/1 -> Gain5/1
  Constant/1 -> Sum/2

== system UAV_formacao/UAV follow/Sensores/inversor r ==
  In1 : Inport
  Constant : Constant  Value=-1250/3
  Gain3 : Gain  Gain=(300-(-300))/(4.3-0.7)
  Gain5 : Gain  Gain=pi/180
  Sum : Sum  Inputs=|++
  Out1 : Outport
  wires:
  In1/1 -> Gain3/1
  Gain5/1 -> Out1/1
  Gain3/1 -> Sum/1
  Sum/1 -> Gain5/1
  Constant/1 -> Sum/2

== system UAV_formacao/UAV follow/Sensores/sensor ==
  beta : Inport
  phi : Inport  Port=2
  lambda : Inport  Port=3
  Constant : Constant  Value=H
  Constant1 : Constant  Value=0
  Constant2 : Constant  Value=0
  MATLAB Function : MATLAB Function  TreatAsAtomicUnit=on
  Mux : Mux  Inputs=3
  Product : Product  Multiplication=Matrix(*)
  Subsystem : Subsystem
  Out1 : Outport
  S : Outport  Port=2
  wires:
  phi/1 -> Subsystem/2(phi_in)
  beta/1 -> Subsystem/3(beta)
  lambda/1 -> Subsystem/1(lambda)
  Subsystem/1(tt) -> MATLAB Function/1(theta)
  Subsystem/2(phi) -> MATLAB Function/2(phi)
  Subsystem/3(psi) -> MATLAB Function/3(psi)
  Constant/1 -> Mux/1
  Constant1/1 -> Mux/2
  Constant2/1 -> Mux/3
  MATLAB Function/1(S) -> Product/1, S/1
  Mux/1 -> Product/2
  Product/1 -> Out1/1

== system UAV_formacao/UAV follow/Sensores/sensor p ==
  r : Inport
  Band-Limited White Noise : simulink/Sources/Band-Limited White Noise  Cov=[sample_time*(4.4)^2]  Ts=sample_time  seed=[9]
  Constant : Constant  Value=2.5
  Gain : Gain  Gain=180/pi
  Gain1 : Gain  Gain=(4.3-0.7)/600
  Saturation : Saturate  UpperLimit=300  LowerLimit=-300
  Sum : Sum  Inputs=|++
  Sum3 : Sum  Inputs=|++
  Out1 : Outport
  wires:
  Gain1/1 -> Sum/1
  Constant/1 -> Sum/2
  Saturation/1 -> Out1/1
  Sum/1 -> Saturation/1
  Band-Limited White Noise/1 -> Sum3/2
  r/1 -> Gain/1
  Gain/1 -> Sum3/1
  Sum3/1 -> Gain1/1

== system UAV_formacao/UAV follow/Sensores/sensor r ==
  r : Inport
  Band-Limited White Noise : simulink/Sources/Band-Limited White Noise  Cov=[sample_time*(4.4)^2]  Ts=sample_time  seed=[10]
  Constant : Constant  Value=2.5
  Gain : Gain  Gain=180/pi
  Gain1 : Gain  Gain=(4.3-0.7)/600
  Saturation : Saturate  UpperLimit=300  LowerLimit=-300
  Sum : Sum  Inputs=|++
  Sum3 : Sum  Inputs=|++
  Out1 : Outport
  wires:
  Gain1/1 -> Sum/1
  Constant/1 -> Sum/2
  Saturation/1 -> Out1/1
  Sum/1 -> Saturation/1
  Band-Limited White Noise/1 -> Sum3/2
  r/1 -> Gain/1
  Gain/1 -> Sum3/1
  Sum3/1 -> Gain1/1

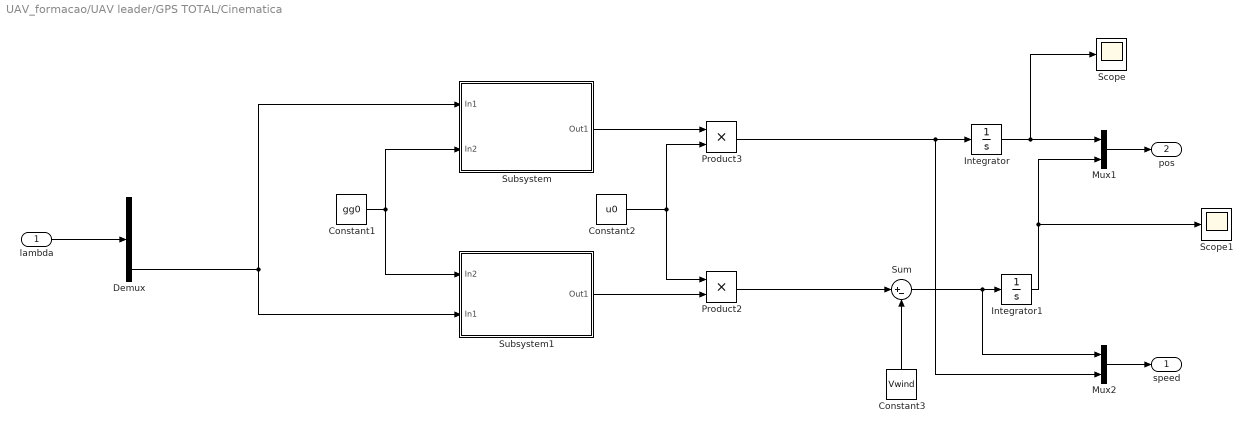
== system UAV_formacao/UAV leader/GPS TOTAL/Cinematica ==
  lambda : Inport
  Constant1 : Constant  Value=gg0
  Constant2 : Constant  Value=u0
  Constant3 : Constant  Value=Vwind
  Demux : Demux  Outputs=5
  Integrator : Integrator  InitialCondition=E0_l
  Integrator1 : Integrator  InitialCondition=N0_l
  Mux1 : Mux  Inputs=2
  Mux2 : Mux  Inputs=2
  Product2 : Product
  Product3 : Product
  Scope : Scope
  Scope1 : Scope
  Subsystem : Subsystem
  Subsystem1 : Subsystem
  Sum : Sum  Inputs=|+-
  speed : Outport
  pos : Outport  Port=2
  wires:
  Constant2/1 -> Product3/2, Product2/1
  Product3/1 -> Mux2/2, Integrator/1
  Product2/1 -> Sum/1
  Constant3/1 -> Sum/2
  Sum/1 -> Mux2/1, Integrator1/1
  Integrator/1 -> Scope/1, Mux1/1
  Mux2/1 -> speed/1
  Mux1/1 -> pos/1
  Subsystem/1(Out1) -> Product3/1
  Constant1/1 -> Subsystem/2(In2), Subsystem1/1(In2)
  Subsystem1/1(Out1) -> Product2/2
  lambda/1 -> Demux/1
  Demux/5 -> Subsystem/1(In1), Subsystem1/2(In1)
  Integrator1/1 -> Scope1/1, Mux1/2

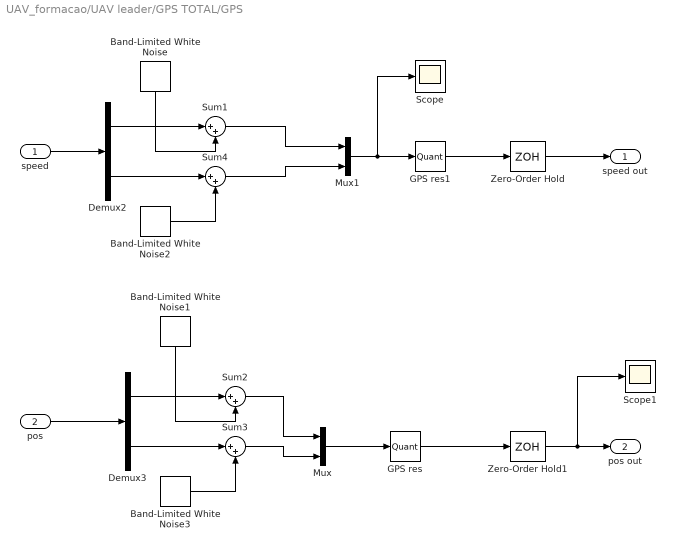
== system UAV_formacao/UAV leader/GPS TOTAL/GPS ==
  speed : Inport
  pos : Inport  Port=2
  Band-Limited White Noise : simulink/Sources/Band-Limited White Noise  Cov=sample_time_gps*0.1*0.1  Ts=sample_time_gps  seed=[5]
  Band-Limited White Noise1 : simulink/Sources/Band-Limited White Noise  Cov=sample_time_gps*2.5*2.5  Ts=sample_time_gps  seed=[7]
  Band-Limited White Noise2 : simulink/Sources/Band-Limited White Noise  Cov=sample_time_gps*0.1*0.1  Ts=sample_time_gps  seed=[6]
  Band-Limited White Noise3 : simulink/Sources/Band-Limited White Noise  Cov=sample_time_gps*2.5*2.5  Ts=sample_time_gps  seed=[8]
  Demux2 : Demux  Outputs=2
  Demux3 : Demux  Outputs=2
  GPS res : Quantizer
  GPS res1 : Quantizer  QuantizationInterval=0.01
  Mux : Mux  Inputs=2
  Mux1 : Mux  Inputs=2
  Scope : Scope
  Scope1 : Scope
  Sum{1..4} (4 alike) : Sum  Inputs=|++
  Zero-Order Hold : ZeroOrderHold  SampleTime=sample_time_gps
  Zero-Order Hold1 : ZeroOrderHold  SampleTime=sample_time_gps
  speed out : Outport
  pos out : Outport  Port=2
  wires:
  Mux/1 -> GPS res/1
  GPS res/1 -> Zero-Order Hold1/1
  GPS res1/1 -> Zero-Order Hold/1
  Mux1/1 -> Scope/1, GPS res1/1
  speed/1 -> Demux2/1
  Demux2/1 -> Sum1/1
  Demux2/2 -> Sum4/1
  Band-Limited White Noise/1 -> Sum1/2
  Band-Limited White Noise2/1 -> Sum4/2
  Demux3/2 -> Sum3/1
  pos/1 -> Demux3/1
  Band-Limited White Noise3/1 -> Sum3/2
  Demux3/1 -> Sum2/1
  Band-Limited White Noise1/1 -> Sum2/2
  Sum2/1 -> Mux/1
  Sum3/1 -> Mux/2
  Sum4/1 -> Mux1/2
  Sum1/1 -> Mux1/1
  Zero-Order Hold/1 -> speed out/1
  Zero-Order Hold1/1 -> Scope1/1, pos out/1

== system UAV_formacao/UAV leader/Sensores/Subsystem ==
  In1 : Inport
  Band-Limited White Noise : simulink/Sources/Band-Limited White Noise  Cov=[sample_time*(2*(5/(2^12)))^2]  Ts=sample_time  seed=[1]
  Quantizer : Quantizer  QuantizationInterval=5/(2^12)
  Saturation : Saturate  UpperLimit=5  LowerLimit=0
  Sum : Sum  Inputs=|++
  Out1 : Outport
  wires:
  In1/1 -> Sum/1
  Saturation/1 -> Out1/1
  Band-Limited White Noise/1 -> Sum/2
  Quantizer/1 -> Saturation/1
  Sum/1 -> Quantizer/1

== system UAV_formacao/UAV leader/Sensores/Subsystem1 ==
  In1 : Inport
  Band-Limited White Noise : simulink/Sources/Band-Limited White Noise  Cov=[sample_time*(2*(5/(2^12)))^2]  Ts=sample_time  seed=[2]
  Quantizer : Quantizer  QuantizationInterval=5/(2^12)
  Saturation : Saturate  UpperLimit=5  LowerLimit=0
  Sum : Sum  Inputs=|++
  Out1 : Outport
  wires:
  In1/1 -> Sum/1
  Saturation/1 -> Out1/1
  Band-Limited White Noise/1 -> Sum/2
  Quantizer/1 -> Saturation/1
  Sum/1 -> Quantizer/1

== system UAV_formacao/UAV leader/Sensores/inversor ==
  In1 : Inport
  Band-Limited White Noise1 : simulink/Sources/Band-Limited White Noise  Cov=[0.005*0.005*freq_amost]  Ts=freq_amost  seed=[3]
  Band-Limited White Noise2 : simulink/Sources/Band-Limited White Noise  Cov=[0.005*0.005*sample_time]  Ts=sample_time  seed=[4]
  Demux : Demux  Outputs=3
  Gain : Gain  Gain=-1
  Quantizer : Quantizer  QuantizationInterval=0.005
  Quantizer1 : Quantizer  QuantizationInterval=0.005
  Saturation : Saturate  UpperLimit=8  LowerLimit=-8
  Saturation1 : Saturate  UpperLimit=8  LowerLimit=-8
  Sum : Sum  Inputs=|++
  Sum1 : Sum  Inputs=|++
  Trigonometric Function : Trigonometry  Operator=atan2
  Out1 : Outport
  wires:
  Band-Limited White Noise1/1 -> Sum/2
  Sum1/1 -> Saturation1/1
  Sum/1 -> Saturation/1
  Band-Limited White Noise2/1 -> Sum1/2
  Saturation/1 -> Quantizer/1
  Saturation1/1 -> Quantizer1/1
  Demux/1 -> Sum/1
  Quantizer1/1 -> Gain/1
  Quantizer/1 -> Trigonometric Function/2
  Trigonometric Function/1 -> Out1/1
  In1/1 -> Demux/1
  Demux/2 -> Sum1/1
  Gain/1 -> Trigonometric Function/1

== system UAV_formacao/UAV leader/Sensores/inversor p ==
  In1 : Inport
  Constant : Constant  Value=-1250/3
  Gain3 : Gain  Gain=(300-(-300))/(4.3-0.7)
  Gain5 : Gain  Gain=pi/180
  Sum : Sum  Inputs=|++
  Out1 : Outport
  wires:
  In1/1 -> Gain3/1
  Gain5/1 -> Out1/1
  Gain3/1 -> Sum/1
  Sum/1 -> Gain5/1
  Constant/1 -> Sum/2

== system UAV_formacao/UAV leader/Sensores/inversor r ==
  In1 : Inport
  Constant : Constant  Value=-1250/3
  Gain3 : Gain  Gain=(300-(-300))/(4.3-0.7)
  Gain5 : Gain  Gain=pi/180
  Sum : Sum  Inputs=|++
  Out1 : Outport
  wires:
  In1/1 -> Gain3/1
  Gain5/1 -> Out1/1
  Gain3/1 -> Sum/1
  Sum/1 -> Gain5/1
  Constant/1 -> Sum/2

== system UAV_formacao/UAV leader/Sensores/sensor ==
  beta : Inport
  phi : Inport  Port=2
  lambda : Inport  Port=3
  Constant : Constant  Value=H
  Constant1 : Constant  Value=0
  Constant2 : Constant  Value=0
  MATLAB Function : MATLAB Function  TreatAsAtomicUnit=on
  Mux : Mux  Inputs=3
  Product : Product  Multiplication=Matrix(*)
  Subsystem : Subsystem
  Out1 : Outport
  wires:
  phi/1 -> Subsystem/2(phi_in)
  beta/1 -> Subsystem/3(beta)
  lambda/1 -> Subsystem/1(lambda)
  Subsystem/1(tt) -> MATLAB Function/1(theta)
  Subsystem/2(phi) -> MATLAB Function/2(phi)
  Subsystem/3(psi) -> MATLAB Function/3(psi)
  Constant/1 -> Mux/1
  Constant1/1 -> Mux/2
  Constant2/1 -> Mux/3
  MATLAB Function/1(S) -> Product/1
  Mux/1 -> Product/2
  Product/1 -> Out1/1

== system UAV_formacao/UAV leader/Sensores/sensor p ==
  r : Inport
  Band-Limited White Noise : simulink/Sources/Band-Limited White Noise  Cov=[sample_time*(4.4)^2]  Ts=sample_time  seed=[1]
  Constant : Constant  Value=2.5
  Gain : Gain  Gain=180/pi
  Gain1 : Gain  Gain=(4.3-0.7)/600
  Saturation : Saturate  UpperLimit=300  LowerLimit=-300
  Sum : Sum  Inputs=|++
  Sum3 : Sum  Inputs=|++
  Out1 : Outport
  wires:
  Gain1/1 -> Sum/1
  Constant/1 -> Sum/2
  Saturation/1 -> Out1/1
  Sum/1 -> Saturation/1
  Band-Limited White Noise/1 -> Sum3/2
  r/1 -> Gain/1
  Gain/1 -> Sum3/1
  Sum3/1 -> Gain1/1

== system UAV_formacao/UAV leader/Sensores/sensor r ==
  r : Inport
  Band-Limited White Noise : simulink/Sources/Band-Limited White Noise  Cov=[sample_time*(4.4)^2]  Ts=sample_time  seed=[2]
  Constant : Constant  Value=2.5
  Gain : Gain  Gain=180/pi
  Gain1 : Gain  Gain=(4.3-0.7)/600
  Saturation : Saturate  UpperLimit=300  LowerLimit=-300
  Sum : Sum  Inputs=|++
  Sum3 : Sum  Inputs=|++
  Out1 : Outport
  wires:
  Gain1/1 -> Sum/1
  Constant/1 -> Sum/2
  Saturation/1 -> Out1/1
  Sum/1 -> Saturation/1
  Band-Limited White Noise/1 -> Sum3/2
  r/1 -> Gain/1
  Gain/1 -> Sum3/1
  Sum3/1 -> Gain1/1

== system UAV_formacao/UAV follow/GPS TOTAL/Cinematica/Subsystem ==
  In1 : Inport
  In2 : Inport  Port=2
  Product : Product
  Trigonometric Function : Trigonometry  Operator=cos
  Trigonometric Function3 : Trigonometry
  Out1 : Outport
  wires:
  Trigonometric Function3/1 -> Product/1
  Trigonometric Function/1 -> Product/2
  In1/1 -> Trigonometric Function3/1
  Product/1 -> Out1/1
  In2/1 -> Trigonometric Function/1

== system UAV_formacao/UAV follow/GPS TOTAL/Cinematica/Subsystem1 ==
  In2 : Inport
  In1 : Inport  Port=2
  Product1 : Product
  Trigonometric Function1 : Trigonometry  Operator=cos
  Trigonometric Function2 : Trigonometry  Operator=cos
  Out1 : Outport
  wires:
  Trigonometric Function2/1 -> Product1/2
  Trigonometric Function1/1 -> Product1/1
  In2/1 -> Trigonometric Function1/1
  In1/1 -> Trigonometric Function2/1
  Product1/1 -> Out1/1

== system UAV_formacao/UAV follow/Sensores/sensor/Subsystem ==
  lambda : Inport
  phi_in : Inport  Port=2
  beta : Inport  Port=3
  Constant : Constant  Value=tt0
  Sum : Sum  Inputs=|+-
  tt : Outport
  phi : Outport  Port=2
  psi : Outport  Port=3
  wires:
  Sum/1 -> psi/1
  Constant/1 -> tt/1
  beta/1 -> Sum/2
  lambda/1 -> Sum/1
  phi_in/1 -> phi/1

== system UAV_formacao/UAV leader/GPS TOTAL/Cinematica/Subsystem ==
  In1 : Inport
  In2 : Inport  Port=2
  Product : Product
  Trigonometric Function : Trigonometry  Operator=cos
  Trigonometric Function3 : Trigonometry
  Out1 : Outport
  wires:
  Trigonometric Function3/1 -> Product/1
  Trigonometric Function/1 -> Product/2
  In1/1 -> Trigonometric Function3/1
  Product/1 -> Out1/1
  In2/1 -> Trigonometric Function/1

== system UAV_formacao/UAV leader/GPS TOTAL/Cinematica/Subsystem1 ==
  In2 : Inport
  In1 : Inport  Port=2
  Product1 : Product
  Trigonometric Function1 : Trigonometry  Operator=cos
  Trigonometric Function2 : Trigonometry  Operator=cos
  Out1 : Outport
  wires:
  Trigonometric Function2/1 -> Product1/2
  Trigonometric Function1/1 -> Product1/1
  In2/1 -> Trigonometric Function1/1
  In1/1 -> Trigonometric Function2/1
  Product1/1 -> Out1/1

== system UAV_formacao/UAV leader/Sensores/sensor/Subsystem ==
  lambda : Inport
  phi_in : Inport  Port=2
  beta : Inport  Port=3
  Constant : Constant  Value=tt0
  Sum : Sum  Inputs=|+-
  tt : Outport
  phi : Outport  Port=2
  psi : Outport  Port=3
  wires:
  Sum/1 -> psi/1
  Constant/1 -> tt/1
  beta/1 -> Sum/2
  lambda/1 -> Sum/1
  phi_in/1 -> phi/1

== matlab function UAV_formacao/UAV leader/Sensores/sensor/MATLAB Function ==
  data: theta input; S output; phi input; psi input
function S = matriz_rotacao(theta, phi, psi)
    
S_phi = [1, 0, 0;
        0, cos(phi), sin(phi);
        0, -sin(phi), cos(phi);];

S_theta = [cos(theta), 0, -sin(theta);
          0, 1, 0;
          sin(theta), 0, cos(theta);];

S_psi = [cos(psi), sin(psi), 0;
        -sin(psi), cos(psi), 0;
        0, 0, 1;];

S = S_phi * S_theta * S_psi;
end

== matlab function UAV_formacao/UAV follow/Sensores/sensor/MATLAB Function ==
  data: theta input; S output; phi input; psi input
function S = matriz_rotacao(theta, phi, psi)
    
S_phi = [1, 0, 0;
        0, cos(phi), sin(phi);
        0, -sin(phi), cos(phi);];

S_theta = [cos(theta), 0, -sin(theta);
          0, 1, 0;
          sin(theta), 0, cos(theta);];

S_psi = [cos(psi), sin(psi), 0;
        -sin(psi), cos(psi), 0;
        0, 0, 1;];

S = S_phi * S_theta * S_psi;
end
